simulink library "dspparest3"  (Simulink 6.0)
values from neighbouring files (symbols this model uses):
  D = D + B    [rebuffer_delay.m]
libraries: dspmtrx3 x22, dspsigattribs x11, simulink x7, dspindex x4, dspsolvers x3, dspstat3 x1
settings Model: RequirementInfo=9  CovMetricSettings=d  Creator=don  LastModifiedBy=sconahan  ExtModeAutoUpdateStatusClock=off

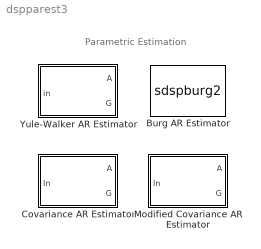
== system dspparest3 ==
  note: Parametric Estimation
  Burg AR Estimator : S-Function  FunctionName=sdspburg2  Parameters=fcn, inheritOrder, ord  mask(Burg AR Estimator){fcn=A, inheritOrder=on, ord=4}
      mask prompts: fcn "Output(s):"; inheritOrder "Inherit estimation order from input dimensions"; ord "Estimation order:"
      mask help: Frame-based parametric AR estimation using the Burg maximum entropy method. Outputs AR model coefficients A and/or reflection coefficients K, plus the model gain, G.
      mask init:
      | s = dspblkburg2('icon');
      mask Help: web(dspbhelp);
      mask StyleString: popup(A and K|A|K),checkbox,edit
      mask CallbackString: |dspblkburg2|
      mask Display:
      | disp('Burg AR\nEstimator');
      | port_label('output',s.o1,s.o1s);
      | port_label('output',s.o2,s.o2s);
      | port_label('output',s.o3,s.o3s);
  Covariance AR Estimator : Subsystem  mask(Covariance AR Estimator){P=4}
      mask prompts: P "Estimation order:"
      mask help: Frame-based parametric AR estimation using the Covariance method. The AR model coefficients are given in A and the gain is given in G.
      mask Help: web(dspbhelp);
      mask Display: disp('Cov AR\nEstimator')
  Modified Covariance AR Estimator : Subsystem  mask(Modified Covariance AR Estimator){P=4}
      mask prompts: P "Estimation order:"
      mask help: Frame-based parametric AR estimation using the Modified Covariance method. The AR model coefficients are given in A and the gain is given in G.
      mask Help: web(dspbhelp);
      mask Display: disp('MCov AR\nEstimator')
  Yule-Walker AR Estimator : Subsystem  mask(Yule-Walker AR Estimator){ywArOutType=A, inheritOrder=on, ord=4}
      mask prompts: ywArOutType "Output(s):"; inheritOrder "Inherit estimation order from input dimensions"; ord "Estimation order:"
      mask help: Frame-based parametric AR estimation using the Yule-Walker method. The AR model coefficients are given in A (polynomial coefficients) and/or K (reflection coefficients). The square of the model gain is given in G.
      mask init:
      | acf = dspblkywestim('computeVars',ord);
      | dspblkywestim('init');
      mask Help: web(dspbhelp);
      mask StyleString: popup(A and K|A|K),checkbox,edit
      mask CallbackString: |dspblkywestim|
      mask Display: disp('Yule AR\nEstimator')

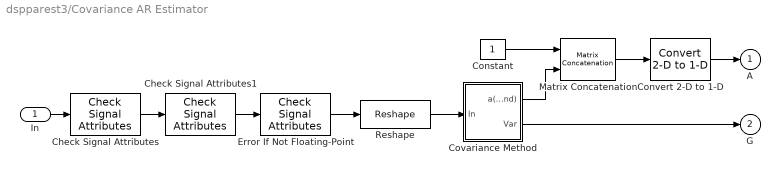
== system dspparest3/Covariance AR Estimator ==
  In : Inport
  Check Signal Attributes : dspsigattribs/Check Signal Attributes  SigAttribCheckMethod=Matches attributes exactly  Complexity=Ignore  Frame=Frame-based  DimsCheckMethod=Is...  Dimensions=Row vector (2-D)  DatatypeCheckMethod=Ignore  DatatypeGeneral=Boolean  DtypeFloatSpecific=Any floating-point  DtypeFixedSpecific=Any fixed-point  DtypeIntSpecific=Any integer  SampleMode=Ignore
  Check Signal Attributes1 : dspsigattribs/Check Signal Attributes  SigAttribCheckMethod=Does not match attributes exactly  Complexity=Ignore  Frame=Ignore  DimsCheckMethod=Is...  Dimensions=Vector (1-D or 2-D)  DatatypeCheckMethod=Ignore  DatatypeGeneral=Boolean  DtypeFloatSpecific=Any floating-point  DtypeFixedSpecific=Any fixed-point  DtypeIntSpecific=Any integer  SampleMode=Ignore
  Constant : Constant
  Convert 2-D to 1-D : dspsigattribs/Convert 2-D to 1-D
  Covariance Method : Subsystem
  Error If Not Floating-Point : dspsigattribs/Check Signal Attributes  SigAttribCheckMethod=Does not match attributes exactly  Complexity=Ignore  Frame=Ignore  DimsCheckMethod=Ignore  Dimensions=1-D  DatatypeCheckMethod=Is...  DatatypeGeneral=Floating-point  DtypeFloatSpecific=Any floating-point  DtypeFixedSpecific=Any fixed-point  DtypeIntSpecific=Any integer  SampleMode=Ignore
  Matrix Concatenation : simulink/Math Operations/Matrix Concatenation  numInports=2  catMethod=Vertical
  Reshape : simulink/Math Operations/Reshape  OutputDimensionality=Column vector  OutputDimensions=[1,1]
  A : Outport  InitialOutput=0
  G : Outport  Port=2  InitialOutput=0
  wires:
  Matrix Concatenation/1 -> Convert 2-D to 1-D/1
  Covariance Method/1(a(2:end)) -> Matrix Concatenation/2
  Constant/1 -> Matrix Concatenation/1
  Covariance Method/2(Var) -> G/1
  Check Signal Attributes/1 -> Check Signal Attributes1/1
  In/1 -> Check Signal Attributes/1
  Reshape/1 -> Covariance Method/1(In)
  Check Signal Attributes1/1 -> Error If Not Floating-Point/1
  Convert 2-D to 1-D/1 -> A/1
  Error If Not Floating-Point/1 -> Reshape/1

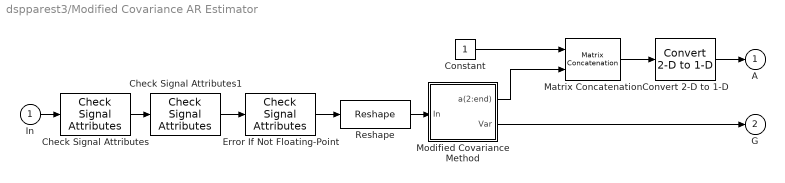
== system dspparest3/Modified Covariance AR Estimator ==
  In : Inport
  Check Signal Attributes : dspsigattribs/Check Signal Attributes  SigAttribCheckMethod=Matches attributes exactly  Complexity=Ignore  Frame=Frame-based  DimsCheckMethod=Is...  Dimensions=Row vector (2-D)  DatatypeCheckMethod=Ignore  DatatypeGeneral=Boolean  DtypeFloatSpecific=Any floating-point  DtypeFixedSpecific=Any fixed-point  DtypeIntSpecific=Any integer  SampleMode=Ignore
  Check Signal Attributes1 : dspsigattribs/Check Signal Attributes  SigAttribCheckMethod=Does not match attributes exactly  Complexity=Ignore  Frame=Ignore  DimsCheckMethod=Is...  Dimensions=Vector (1-D or 2-D)  DatatypeCheckMethod=Ignore  DatatypeGeneral=Boolean  DtypeFloatSpecific=Any floating-point  DtypeFixedSpecific=Any fixed-point  DtypeIntSpecific=Any integer  SampleMode=Ignore
  Constant : Constant
  Convert 2-D to 1-D : dspsigattribs/Convert 2-D to 1-D
  Error If Not Floating-Point : dspsigattribs/Check Signal Attributes  SigAttribCheckMethod=Does not match attributes exactly  Complexity=Ignore  Frame=Ignore  DimsCheckMethod=Ignore  Dimensions=1-D  DatatypeCheckMethod=Is...  DatatypeGeneral=Floating-point  DtypeFloatSpecific=Any floating-point  DtypeFixedSpecific=Any fixed-point  DtypeIntSpecific=Any integer  SampleMode=Ignore
  Matrix Concatenation : simulink/Math Operations/Matrix Concatenation  numInports=2  catMethod=Vertical
  Modified Covariance Method : Subsystem
  Reshape : simulink/Math Operations/Reshape  OutputDimensionality=Column vector  OutputDimensions=[1,1]
  A : Outport  InitialOutput=0
  G : Outport  Port=2  InitialOutput=0
  wires:
  Modified Covariance Method/2(Var) -> G/1
  Constant/1 -> Matrix Concatenation/1
  Matrix Concatenation/1 -> Convert 2-D to 1-D/1
  Modified Covariance Method/1(a(2:end)) -> Matrix Concatenation/2
  In/1 -> Check Signal Attributes/1
  Reshape/1 -> Modified Covariance Method/1(In)
  Check Signal Attributes1/1 -> Error If Not Floating-Point/1
  Check Signal Attributes/1 -> Check Signal Attributes1/1
  Convert 2-D to 1-D/1 -> A/1
  Error If Not Floating-Point/1 -> Reshape/1

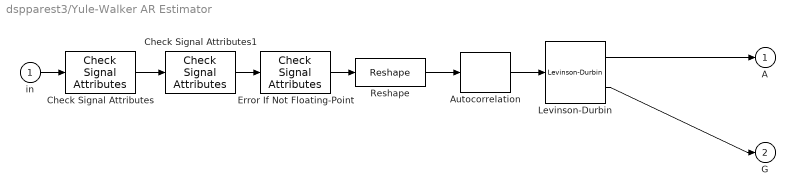
== system dspparest3/Yule-Walker AR Estimator ==
  in : Inport
  Autocorrelation : dspstat3/Autocorrelation  DialogController=dspDDGCreate  DialogControllerArgs=DataTag0  AllPositiveLags=on  maxlag=acf  bias=Biased  domain=Time  roundingMode=Floor  overflowMode=off
  Check Signal Attributes : dspsigattribs/Check Signal Attributes  SigAttribCheckMethod=Matches attributes exactly  Complexity=Ignore  Frame=Frame-based  DimsCheckMethod=Is...  Dimensions=Row vector (2-D)  DatatypeCheckMethod=Ignore  DatatypeGeneral=Boolean  DtypeFloatSpecific=Any floating-point  DtypeFixedSpecific=Any fixed-point  DtypeIntSpecific=Any integer  SampleMode=Ignore
  Check Signal Attributes1 : dspsigattribs/Check Signal Attributes  SigAttribCheckMethod=Does not match attributes exactly  Complexity=Ignore  Frame=Ignore  DimsCheckMethod=Is...  Dimensions=Vector (1-D or 2-D) or scalar  DatatypeCheckMethod=Ignore  DatatypeGeneral=Boolean  DtypeFloatSpecific=Any floating-point  DtypeFixedSpecific=Any fixed-point  DtypeIntSpecific=Any integer  SampleMode=Ignore
  Error If Not Floating-Point : dspsigattribs/Check Signal Attributes  SigAttribCheckMethod=Does not match attributes exactly  Complexity=Ignore  Frame=Ignore  DimsCheckMethod=Ignore  Dimensions=1-D  DatatypeCheckMethod=Is...  DatatypeGeneral=Floating-point  DtypeFloatSpecific=Any floating-point  DtypeFixedSpecific=Any fixed-point  DtypeIntSpecific=Any integer  SampleMode=Ignore
  Levinson-Durbin : dspsolvers/Levinson-Durbin  coeffOutFcn=A  outP=on  zeroInpHandling=on  firstCoeffMode=Binary point scaling  firstCoeffWordLength=16  firstCoeffFracLength=15  secondCoeffMode=Binary point scaling  secondCoeffWordLength=16  secondCoeffFracLength=15  accumMode=User-defined  accumWordLength=32  accumFracLength=30  prodOutputMode=User-defined  prodOutputWordLength=32  prodOutputFracLength=30  roundingMode=Floor  overflowMode=off
      settings: allowOverrides=off
  Reshape : simulink/Math Operations/Reshape  OutputDimensionality=Column vector  OutputDimensions=[1,1]
  A : Outport  InitialOutput=0
  G : Outport  Port=2
  wires:
  Levinson-Durbin/2 -> G/1
  Autocorrelation/1 -> Levinson-Durbin/1
  Levinson-Durbin/1 -> A/1
  in/1 -> Check Signal Attributes/1
  Check Signal Attributes1/1 -> Error If Not Floating-Point/1
  Reshape/1 -> Autocorrelation/1
  Check Signal Attributes/1 -> Check Signal Attributes1/1
  Error If Not Floating-Point/1 -> Reshape/1

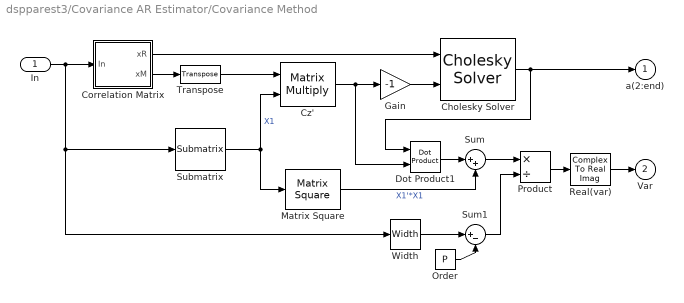
== system dspparest3/Covariance AR Estimator/Covariance Method ==
  In : Inport
  Cholesky Solver : dspsolvers/Cholesky Solver  errmode=Warning
  Correlation Matrix : Subsystem
  Cz' : dspmtrx3/Matrix Multiply  numInputPorts=2  OptimizationLevel=None
  Dot Product1 : simulink/Math Operations/Dot Product  OutDataType=sfix(16)  OutScaling=2^-10  DoSatur=off
  Gain : Gain  Gain=-1  SaturateOnIntegerOverflow=on
  Matrix Square : dspmtrx3/Matrix Square
  Order : Constant  Value=P
  Product : Product  Inputs=*/  SaturateOnIntegerOverflow=on  InputSameDT=on
  Real(var) : ComplexToRealImag  Output=Real
  Submatrix : dspmtrx3/Submatrix  RowSpan=Range of rows  RowStartMode=Index  RowStartIndex=P+1  RowEndMode=Last  RowEndIndex=1  ColSpan=All columns  ColStartMode=First  ColStartIndex=1  ColEndMode=Last  ColEndIndex=1
  Sum : Sum  Inputs=|++  SaturateOnIntegerOverflow=on  InputSameDT=on
  Sum1 : Sum  Inputs=|+-  SaturateOnIntegerOverflow=on  InputSameDT=on
  Transpose : dspmtrx3/Transpose  Hermitian=on  overflowFlag=on
  Width : Width  ShowAdditionalParam=on  OutputDataTypeScalingMode=All ports same datatype
  a(2:end) : Outport  InitialOutput=0
  Var : Outport  Port=2  InitialOutput=0
  wires:
  Order/1 -> Sum1/2
  Width/1 -> Sum1/1
  In/1 -> Correlation Matrix/1(In), Submatrix/1, Width/1
  Cz'/1 -> Dot Product1/2, Gain/1
  Submatrix/1 -> Cz'/2, Matrix Square/1  "X1"
  Correlation Matrix/2(xM) -> Transpose/1
  Transpose/1 -> Cz'/1
  Gain/1 -> Cholesky Solver/2
  Correlation Matrix/1(xR) -> Cholesky Solver/1
  Cholesky Solver/1 -> Dot Product1/1, a(2:end)/1
  Dot Product1/1 -> Sum/1
  Matrix Square/1 -> Sum/2  "X1'*X1"
  Sum/1 -> Product/1
  Product/1 -> Real(var)/1
  Real(var)/1 -> Var/1
  Sum1/1 -> Product/2

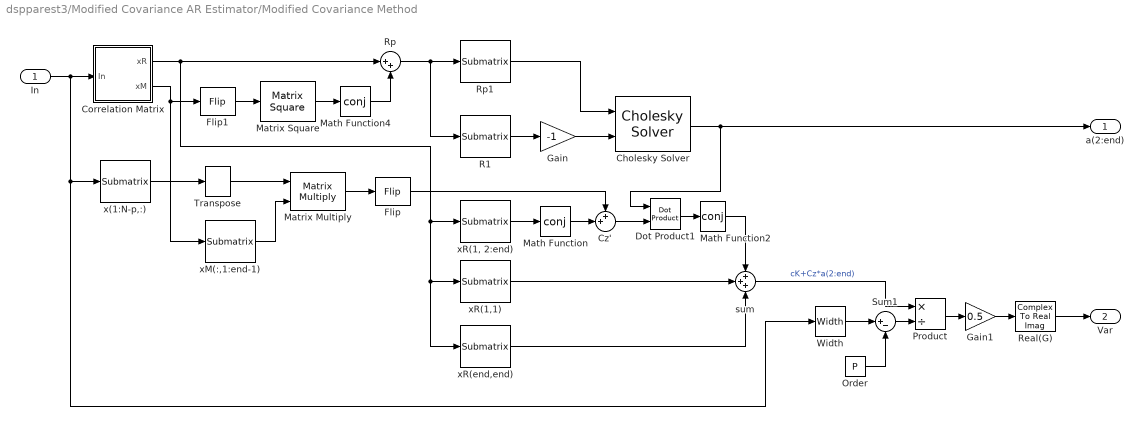
== system dspparest3/Modified Covariance AR Estimator/Modified Covariance Method ==
  In : Inport
  Cholesky Solver : dspsolvers/Cholesky Solver  errmode=Warning
  Correlation Matrix : Subsystem
  Cz' : Sum  Inputs=++|  SaturateOnIntegerOverflow=on  InputSameDT=on
  Dot Product1 : simulink/Math Operations/Dot Product  OutDataType=sfix(16)  OutScaling=2^-10  DoSatur=off
  Flip : dspindex/Flip  dim=Rows
  Flip1 : dspindex/Flip  dim=Rows
  Gain : Gain  Gain=-1  SaturateOnIntegerOverflow=on
  Gain1 : Gain  Gain=0.5  SaturateOnIntegerOverflow=on
  Math Function : Math  Operator=conj  SaturateOnIntegerOverflow=on
  Math Function2 : Math  Operator=conj  SaturateOnIntegerOverflow=on
  Math Function4 : Math  Operator=conj  SaturateOnIntegerOverflow=on
  Matrix Square : dspmtrx3/Matrix Square
  Matrix Multiply : dspmtrx3/Matrix Multiply  numInputPorts=2  OptimizationLevel=None
  Order : Constant  Value=P
  Product : Product  Inputs=*/  SaturateOnIntegerOverflow=on  InputSameDT=on
  R1 : dspmtrx3/Submatrix  RowSpan=Range of rows  RowStartMode=Index  RowStartIndex=2  RowEndMode=Last  RowEndIndex=P  ColSpan=One column  ColStartMode=First  ColStartIndex=2  ColEndMode=Last  ColEndIndex=1
  Real(G) : ComplexToRealImag  Output=Real
  Rp : Sum  Inputs=|++  SaturateOnIntegerOverflow=on  InputSameDT=on
  Rp1 : dspmtrx3/Submatrix  RowSpan=Range of rows  RowStartMode=Index  RowStartIndex=2  RowEndMode=Last  RowEndIndex=P  ColSpan=Range of columns  ColStartMode=Index  ColStartIndex=2  ColEndMode=Last  ColEndIndex=1
  Sum1 : Sum  Inputs=|+-  SaturateOnIntegerOverflow=on  InputSameDT=on
  Transpose : dspmtrx3/Transpose  Hermitian=on  overflowFlag=on
  Width : Width  ShowAdditionalParam=on  OutputDataTypeScalingMode=All ports same datatype
  sum : Sum  Inputs=+++  SaturateOnIntegerOverflow=on  InputSameDT=on
  x(1:N-p,:) : dspmtrx3/Submatrix  RowSpan=Range of rows  RowStartMode=First  RowStartIndex=1  RowEndMode=Offset from last  RowEndIndex=P  ColSpan=All columns  ColStartMode=First  ColStartIndex=1  ColEndMode=Index  ColEndIndex=P
  xM(:,1:end-1) : dspmtrx3/Submatrix  RowSpan=All rows  RowStartMode=First  RowStartIndex=1  RowEndMode=Offset from last  RowEndIndex=P  ColSpan=Range of columns  ColStartMode=First  ColStartIndex=1  ColEndMode=Offset from last  ColEndIndex=1
  "xR(1, 2:end)" : dspmtrx3/Submatrix  RowSpan=One row  RowStartMode=First  RowStartIndex=2  RowEndMode=Last  RowEndIndex=P  ColSpan=Range of columns  ColStartMode=Index  ColStartIndex=2  ColEndMode=Last  ColEndIndex=1
  xR(1,1) : dspmtrx3/Submatrix  RowSpan=One row  RowStartMode=First  RowStartIndex=2  RowEndMode=Index  RowEndIndex=1  ColSpan=One column  ColStartMode=First  ColStartIndex=2  ColEndMode=Last  ColEndIndex=1
  xR(end,end) : dspmtrx3/Submatrix  RowSpan=One row  RowStartMode=Last  RowStartIndex=0  RowEndMode=Last  RowEndIndex=1  ColSpan=One column  ColStartMode=Last  ColStartIndex=0  ColEndMode=Last  ColEndIndex=1
  a(2:end) : Outport
  Var : Outport  Port=2
  wires:
  sum/1 -> Product/1  "cK+Cz*a(2:end)"
  Product/1 -> Gain1/1
  Order/1 -> Sum1/2
  Width/1 -> Sum1/1
  Sum1/1 -> Product/2
  Correlation Matrix/1(xR) -> "xR(1, 2:end)"/1, xR(1,1)/1, xR(end,end)/1, Rp/1
  In/1 -> Correlation Matrix/1(In), Width/1, x(1:N-p,:)/1
  Math Function4/1 -> Rp/2
  Flip1/1 -> Matrix Square/1
  xM(:,1:end-1)/1 -> Matrix Multiply/2
  Math Function/1 -> Cz'/2
  "xR(1, 2:end)"/1 -> Math Function/1
  Flip/1 -> Cz'/1
  Matrix Multiply/1 -> Flip/1
  Dot Product1/1 -> Math Function2/1
  Cz'/1 -> Dot Product1/2
  Matrix Square/1 -> Math Function4/1
  Correlation Matrix/2(xM) -> xM(:,1:end-1)/1, Flip1/1
  Transpose/1 -> Matrix Multiply/1
  x(1:N-p,:)/1 -> Transpose/1
  Rp/1 -> Rp1/1, R1/1
  Cholesky Solver/1 -> a(2:end)/1, Dot Product1/1
  R1/1 -> Gain/1
  Gain/1 -> Cholesky Solver/2
  xR(1,1)/1 -> sum/2
  xR(end,end)/1 -> sum/3
  Math Function2/1 -> sum/1
  Gain1/1 -> Real(G)/1
  Real(G)/1 -> Var/1
  Rp1/1 -> Cholesky Solver/1

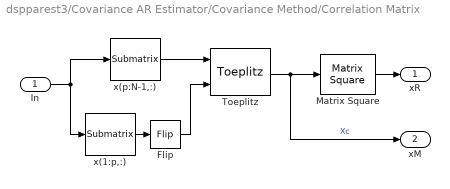
== system dspparest3/Covariance AR Estimator/Covariance Method/Correlation Matrix ==
  In : Inport
  Flip : dspindex/Flip  dim=Columns
  Matrix Square : dspmtrx3/Matrix Square
  Toeplitz : dspmtrx3/Toeplitz  Symmetric=off
  x(1:p,:) : dspmtrx3/Submatrix  RowSpan=Range of rows  RowStartMode=First  RowStartIndex=P  RowEndMode=Index  RowEndIndex=P  ColSpan=All columns  ColStartMode=First  ColStartIndex=1  ColEndMode=Last  ColEndIndex=1
  x(p:N-1,:) : dspmtrx3/Submatrix  RowSpan=Range of rows  RowStartMode=Index  RowStartIndex=P  RowEndMode=Offset from last  RowEndIndex=1  ColSpan=All columns  ColStartMode=First  ColStartIndex=1  ColEndMode=Last  ColEndIndex=1
  xR : Outport
  xM : Outport  Port=2
  wires:
  x(1:p,:)/1 -> Flip/1
  x(p:N-1,:)/1 -> Toeplitz/1
  Toeplitz/1 -> Matrix Square/1, xM/1  "Xc"
  In/1 -> x(p:N-1,:)/1, x(1:p,:)/1
  Matrix Square/1 -> xR/1
  Flip/1 -> Toeplitz/2

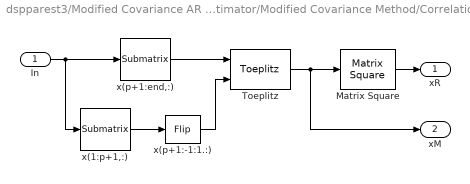
== system dspparest3/Modified Covariance AR Estimator/Modified Covariance Method/Correlation Matrix ==
  In : Inport
  Matrix Square : dspmtrx3/Matrix Square
  Toeplitz : dspmtrx3/Toeplitz  Symmetric=off  overflowFlag=on
  x(1:p+1,:) : dspmtrx3/Submatrix  RowSpan=Range of rows  RowStartMode=First  RowStartIndex=P  RowEndMode=Index  RowEndIndex=P+1  ColSpan=All columns  ColStartMode=First  ColStartIndex=1  ColEndMode=Last  ColEndIndex=1
  x(p+1:-1:1.:) : dspindex/Flip  dim=Columns
  x(p+1:end,:) : dspmtrx3/Submatrix  RowSpan=Range of rows  RowStartMode=Index  RowStartIndex=P+1  RowEndMode=Last  RowEndIndex=1  ColSpan=All columns  ColStartMode=First  ColStartIndex=1  ColEndMode=Last  ColEndIndex=1
  xR : Outport
  xM : Outport  Port=2
  wires:
  x(1:p+1,:)/1 -> x(p+1:-1:1.:)/1
  x(p+1:-1:1.:)/1 -> Toeplitz/2
  Toeplitz/1 -> xM/1, Matrix Square/1
  In/1 -> x(1:p+1,:)/1, x(p+1:end,:)/1
  Matrix Square/1 -> xR/1
  x(p+1:end,:)/1 -> Toeplitz/1
